simulink model "Segway_NL_nuovip"  (R2023b)
settings: Solver=ode1be  StartTime=0.0  StopTime=50  RelTol=1e-3
values from neighbouring files (symbols this model uses):
  dphi_0 = 0    [Parametri_Segway_Simulink_CSI_nuovip.m]
  dtheta_0 = 0    [Parametri_Segway_Simulink_CSI_nuovip.m]
  dx_0 = 0    [Parametri_Segway_Simulink_CSI_nuovip.m]
  Ga_nom_ss = minreal(Ga_nom_ss)    [CSI1_Segway_LQG_nuovip.m]
  K_LQG = -lqgreg(kest, Klqr)    [CSI1_Segway_LQG_nuovip.m]
  phi_0 = 0*pi/180    (= 0)    [Parametri_Segway_Simulink_CSI_nuovip.m]
  theta_0 = 0    [Parametri_Segway_Simulink_CSI_nuovip.m]
  x_0 = 0    [Parametri_Segway_Simulink_CSI_nuovip.m]
undefined symbols (not defined in the file or in its folder): K_DK, K_MS
settings Model: Creator=dario  LastModifiedBy=dario
settings OptimizationCC: ReuseModelBlockBuffer=off

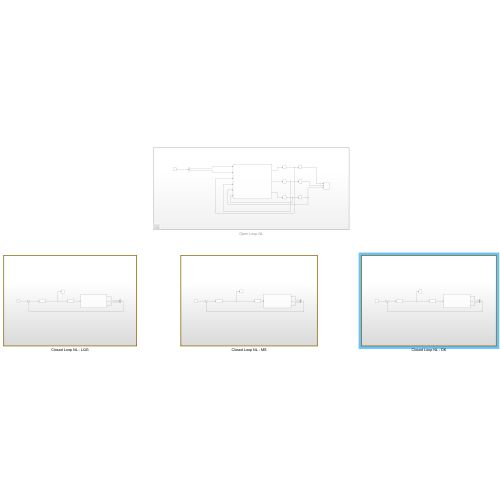
[thumbnail: Simulink's stored preview of the top-level diagram]
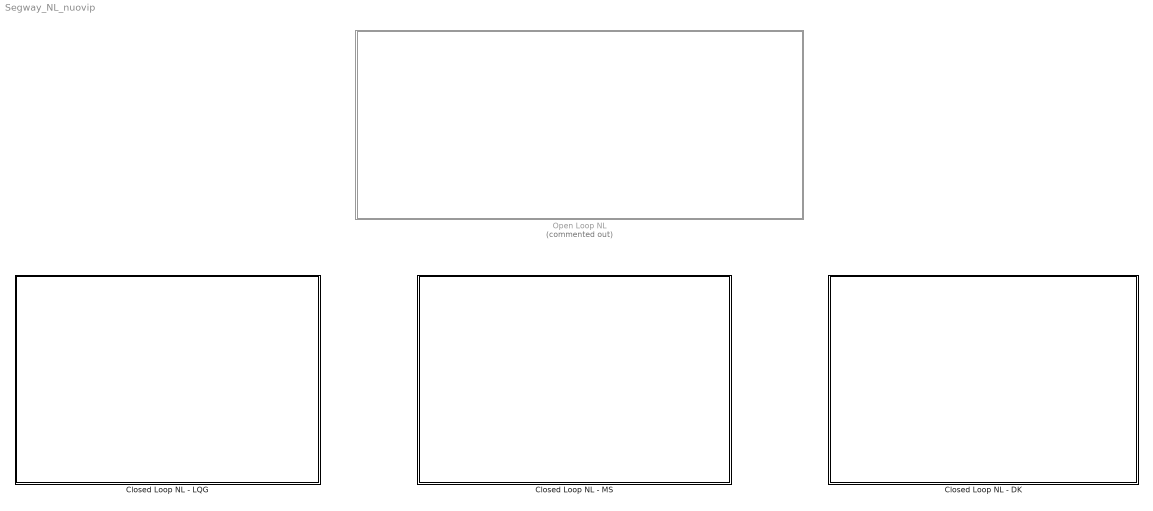
== system Segway_NL_nuovip ==
  Closed Loop NL - DK : Subsystem
  Closed Loop NL - LQG : Subsystem
  Closed Loop NL - MS : Subsystem
  Open Loop NL : Subsystem  Commented=on

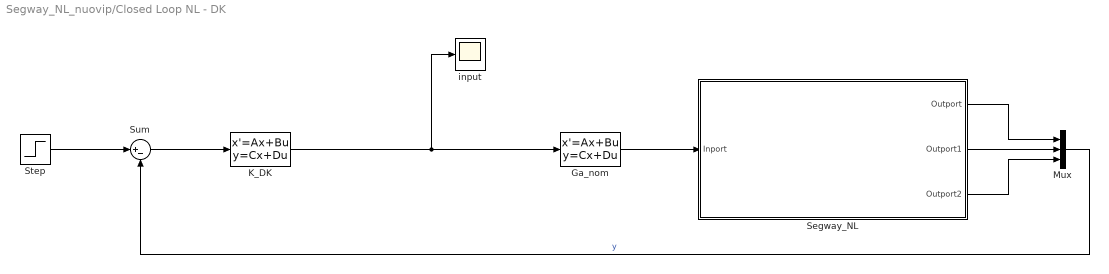
== system Segway_NL_nuovip/Closed Loop NL - DK ==
  Ga_nom : StateSpace  A=Ga_nom_ss.A  B=Ga_nom_ss.B  C=Ga_nom_ss.C  D=Ga_nom_ss.D  InitialCondition=0
  K_DK : StateSpace  A=K_DK.A  B=K_DK.B  C=K_DK.C  D=K_DK.D  InitialCondition=0
  Mux : Mux  Inputs=3
  Segway_NL : Subsystem
  Step : Step  Time=5  Before=[0 0 0]'  After=[0.1 0 0]'  SampleTime=0
  Sum : Sum  Inputs=|+-
  input : Scope
  wires:
  Segway_NL/3(Outport2) -> Mux/3
  K_DK/1 -> Ga_nom/1, input/1
  Step/1 -> Sum/1
  Mux/1 -> Sum/2  "y"
  Ga_nom/1 -> Segway_NL/1(Inport)
  Segway_NL/2(Outport1) -> Mux/2
  Segway_NL/1(Outport) -> Mux/1
  Sum/1 -> K_DK/1

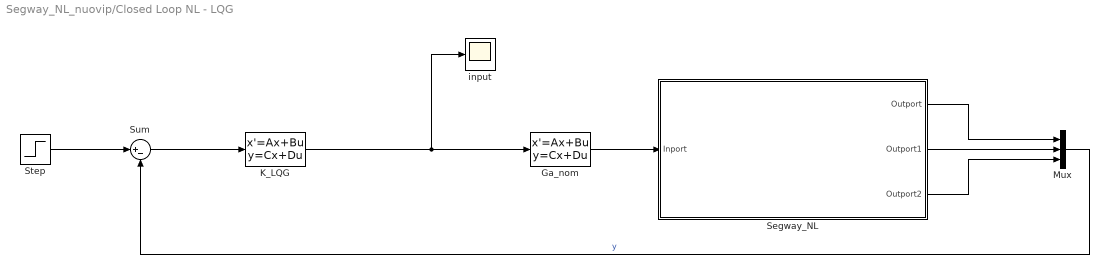
== system Segway_NL_nuovip/Closed Loop NL - LQG ==
  Ga_nom : StateSpace  A=Ga_nom_ss.A  B=Ga_nom_ss.B  C=Ga_nom_ss.C  D=Ga_nom_ss.D  InitialCondition=0
  K_LQG : StateSpace  A=K_LQG.A  B=K_LQG.B  C=K_LQG.C  D=K_LQG.D  InitialCondition=0
  Mux : Mux  Inputs=3
  Segway_NL : Subsystem
  Step : Step  Time=5  Before=[0 0 0]'  After=[10 0 0]'  SampleTime=0
  Sum : Sum  Inputs=|+-
  input : Scope
  wires:
  Segway_NL/3(Outport2) -> Mux/3
  K_LQG/1 -> Ga_nom/1, input/1
  Step/1 -> Sum/1
  Mux/1 -> Sum/2  "y"
  Ga_nom/1 -> Segway_NL/1(Inport)
  Segway_NL/2(Outport1) -> Mux/2
  Segway_NL/1(Outport) -> Mux/1
  Sum/1 -> K_LQG/1

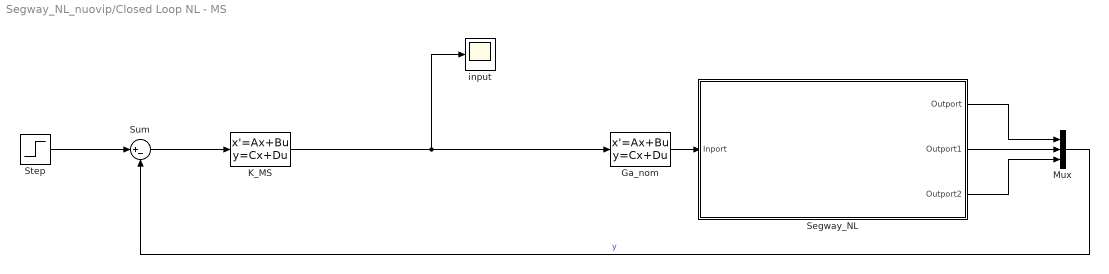
== system Segway_NL_nuovip/Closed Loop NL - MS ==
  Ga_nom : StateSpace  A=Ga_nom_ss.A  B=Ga_nom_ss.B  C=Ga_nom_ss.C  D=Ga_nom_ss.D  InitialCondition=0
  K_MS : StateSpace  A=K_MS.A  B=K_MS.B  C=K_MS.C  D=K_MS.D  InitialCondition=0
  Mux : Mux  Inputs=3
  Segway_NL : Subsystem
  Step : Step  Time=2  Before=[0 0 0]'  After=[50 0 0]'  SampleTime=0
  Sum : Sum  Inputs=|+-
  input : Scope
  wires:
  Sum/1 -> K_MS/1
  Segway_NL/1(Outport) -> Mux/1
  Segway_NL/2(Outport1) -> Mux/2
  Ga_nom/1 -> Segway_NL/1(Inport)
  Mux/1 -> Sum/2  "y"
  Step/1 -> Sum/1
  K_MS/1 -> input/1, Ga_nom/1
  Segway_NL/3(Outport2) -> Mux/3

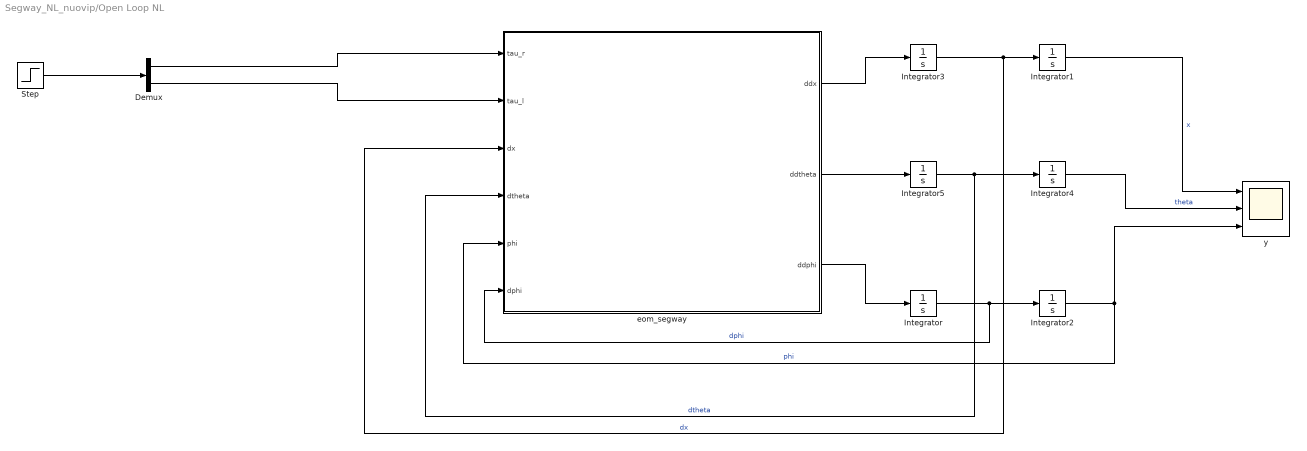
== system Segway_NL_nuovip/Open Loop NL ==
  Demux : Demux  Outputs=2
  Integrator : Integrator  InitialCondition=dphi_0
  Integrator1 : Integrator  InitialCondition=x_0
  Integrator2 : Integrator  InitialCondition=phi_0
  Integrator3 : Integrator  InitialCondition=dx_0
  Integrator4 : Integrator  InitialCondition=theta_0
  Integrator5 : Integrator  InitialCondition=dtheta_0
  Step : Step  Time=5  Before=[0 0]'  After=0.01*[1 1]'  SampleTime=0
  eom_segway : MATLAB Function  TreatAsAtomicUnit=on
  y : Scope  NumInputPorts=3
  wires:
  Integrator1/1 -> y/1  "x"
  Integrator4/1 -> y/2  "theta"
  Integrator5/1 -> eom_segway/4(dtheta), Integrator4/1  "dtheta"
  Demux/1 -> eom_segway/1(tau_r)
  Demux/2 -> eom_segway/2(tau_l)
  eom_segway/3(ddphi) -> Integrator/1
  Integrator3/1 -> eom_segway/3(dx), Integrator1/1  "dx"
  Integrator2/1 -> y/3, eom_segway/5(phi)  "phi"
  eom_segway/1(ddx) -> Integrator3/1
  Integrator/1 -> eom_segway/6(dphi), Integrator2/1  "dphi"
  eom_segway/2(ddtheta) -> Integrator5/1
  Step/1 -> Demux/1

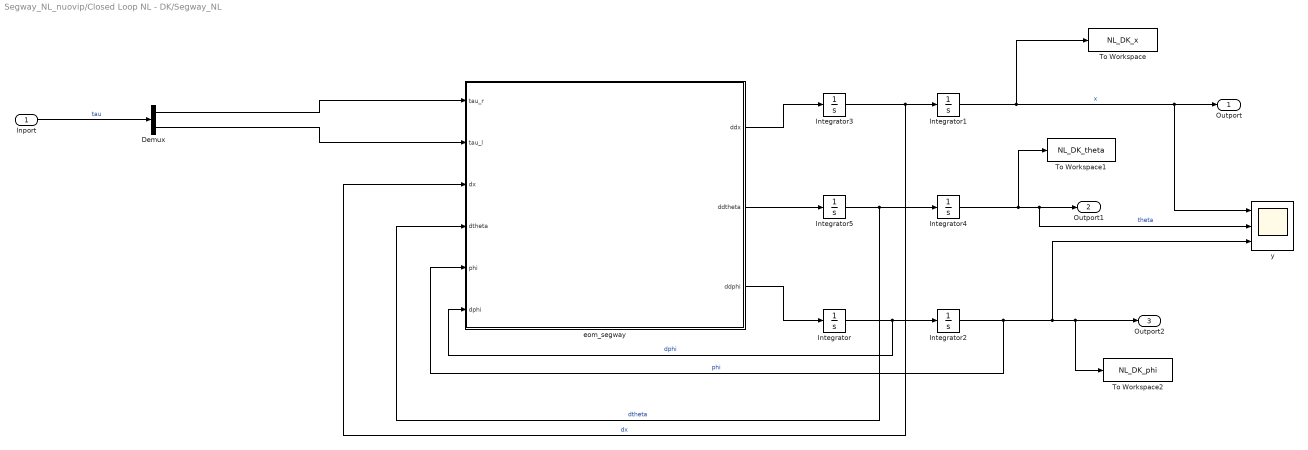
== system Segway_NL_nuovip/Closed Loop NL - DK/Segway_NL ==
  Inport : Inport
  Demux : Demux  Outputs=2
  Integrator : Integrator  InitialCondition=dphi_0
  Integrator1 : Integrator  InitialCondition=x_0
  Integrator2 : Integrator  InitialCondition=phi_0
  Integrator3 : Integrator  InitialCondition=dx_0
  Integrator4 : Integrator  InitialCondition=theta_0
  Integrator5 : Integrator  InitialCondition=dtheta_0
  To Workspace : ToWorkspace  VariableName=NL_DK_x  SaveFormat=Timeseries  SampleTime=-1
  To Workspace1 : ToWorkspace  VariableName=NL_DK_theta  SaveFormat=Timeseries  SampleTime=-1
  To Workspace2 : ToWorkspace  VariableName=NL_DK_phi  SaveFormat=Timeseries  SampleTime=-1
  eom_segway : MATLAB Function  TreatAsAtomicUnit=on
  y : Scope  NumInputPorts=3
  Outport : Outport
  Outport1 : Outport  Port=2
  Outport2 : Outport  Port=3
  wires:
  Integrator1/1 -> To Workspace/1, y/1, Outport/1  "x"
  eom_segway/1(ddx) -> Integrator3/1
  Integrator2/1 -> y/3, To Workspace2/1, Outport2/1, eom_segway/5(phi)  "phi"
  Integrator/1 -> eom_segway/6(dphi), Integrator2/1  "dphi"
  Integrator3/1 -> eom_segway/3(dx), Integrator1/1  "dx"
  eom_segway/3(ddphi) -> Integrator/1
  eom_segway/2(ddtheta) -> Integrator5/1
  Integrator5/1 -> eom_segway/4(dtheta), Integrator4/1  "dtheta"
  Integrator4/1 -> To Workspace1/1, y/2, Outport1/1  "theta"
  Inport/1 -> Demux/1  "tau"
  Demux/1 -> eom_segway/1(tau_r)
  Demux/2 -> eom_segway/2(tau_l)

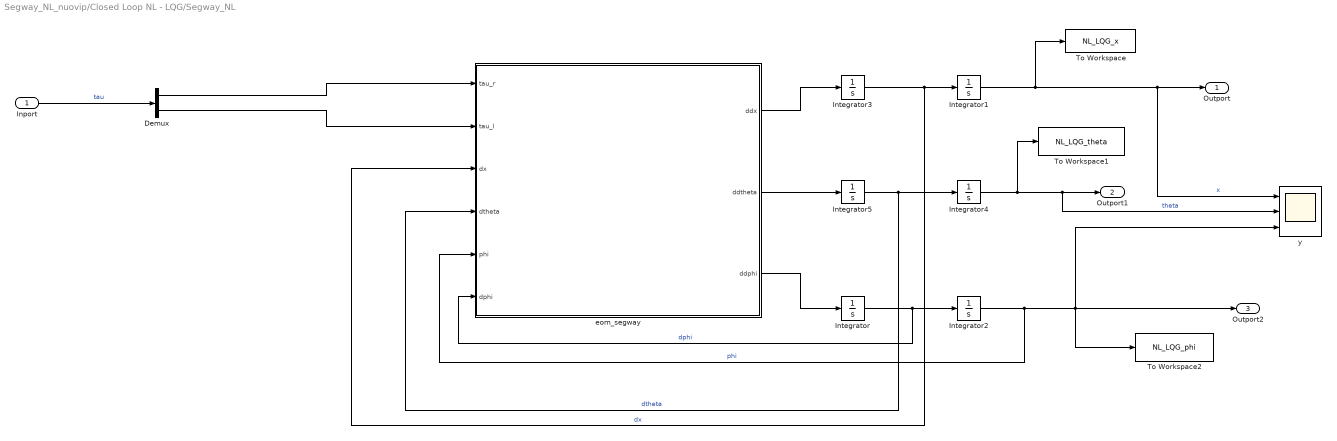
== system Segway_NL_nuovip/Closed Loop NL - LQG/Segway_NL ==
  Inport : Inport
  Demux : Demux  Outputs=2
  Integrator : Integrator  InitialCondition=dphi_0
  Integrator1 : Integrator  InitialCondition=x_0
  Integrator2 : Integrator  InitialCondition=phi_0
  Integrator3 : Integrator  InitialCondition=dx_0
  Integrator4 : Integrator  InitialCondition=theta_0
  Integrator5 : Integrator  InitialCondition=dtheta_0
  To Workspace : ToWorkspace  VariableName=NL_LQG_x  SaveFormat=Timeseries  SampleTime=-1
  To Workspace1 : ToWorkspace  VariableName=NL_LQG_theta  SaveFormat=Timeseries  SampleTime=-1
  To Workspace2 : ToWorkspace  VariableName=NL_LQG_phi  SaveFormat=Timeseries  SampleTime=-1
  eom_segway : MATLAB Function  TreatAsAtomicUnit=on
  y : Scope  NumInputPorts=3
  Outport : Outport
  Outport1 : Outport  Port=2
  Outport2 : Outport  Port=3
  wires:
  Integrator1/1 -> To Workspace/1, y/1, Outport/1  "x"
  eom_segway/1(ddx) -> Integrator3/1
  Integrator2/1 -> To Workspace2/1, y/3, Outport2/1, eom_segway/5(phi)  "phi"
  Integrator/1 -> eom_segway/6(dphi), Integrator2/1  "dphi"
  Integrator3/1 -> eom_segway/3(dx), Integrator1/1  "dx"
  eom_segway/3(ddphi) -> Integrator/1
  eom_segway/2(ddtheta) -> Integrator5/1
  Integrator5/1 -> eom_segway/4(dtheta), Integrator4/1  "dtheta"
  Integrator4/1 -> To Workspace1/1, y/2, Outport1/1  "theta"
  Inport/1 -> Demux/1  "tau"
  Demux/1 -> eom_segway/1(tau_r)
  Demux/2 -> eom_segway/2(tau_l)

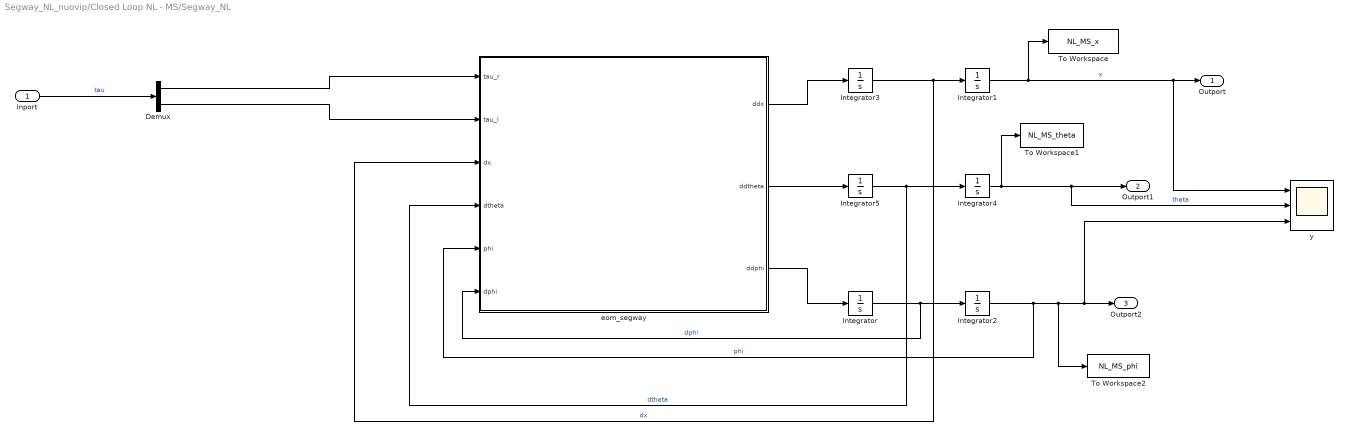
== system Segway_NL_nuovip/Closed Loop NL - MS/Segway_NL ==
  Inport : Inport
  Demux : Demux  Outputs=2
  Integrator : Integrator  InitialCondition=dphi_0
  Integrator1 : Integrator  InitialCondition=x_0
  Integrator2 : Integrator  InitialCondition=phi_0
  Integrator3 : Integrator  InitialCondition=dx_0
  Integrator4 : Integrator  InitialCondition=theta_0
  Integrator5 : Integrator  InitialCondition=dtheta_0
  To Workspace : ToWorkspace  VariableName=NL_MS_x  SaveFormat=Timeseries  SampleTime=-1
  To Workspace1 : ToWorkspace  VariableName=NL_MS_theta  SaveFormat=Timeseries  SampleTime=-1
  To Workspace2 : ToWorkspace  VariableName=NL_MS_phi  SaveFormat=Timeseries  SampleTime=-1
  eom_segway : MATLAB Function  TreatAsAtomicUnit=on
  y : Scope  NumInputPorts=3
  Outport : Outport
  Outport1 : Outport  Port=2
  Outport2 : Outport  Port=3
  wires:
  Demux/2 -> eom_segway/2(tau_l)
  Demux/1 -> eom_segway/1(tau_r)
  Inport/1 -> Demux/1  "tau"
  Integrator4/1 -> To Workspace1/1, Outport1/1, y/2  "theta"
  Integrator5/1 -> Integrator4/1, eom_segway/4(dtheta)  "dtheta"
  eom_segway/2(ddtheta) -> Integrator5/1
  eom_segway/3(ddphi) -> Integrator/1
  Integrator3/1 -> Integrator1/1, eom_segway/3(dx)  "dx"
  Integrator/1 -> Integrator2/1, eom_segway/6(dphi)  "dphi"
  Integrator2/1 -> eom_segway/5(phi), To Workspace2/1, Outport2/1, y/3  "phi"
  eom_segway/1(ddx) -> Integrator3/1
  Integrator1/1 -> To Workspace/1, Outport/1, y/1  "x"

== matlab function Segway_NL_nuovip/Open Loop NL/eom_segway ==
  data: ddx output size=1; ddtheta output; tau_r input; tau_l input; dx input; dtheta input; phi input; dphi input; ddphi output; eom_params parameter
% function that describes the EoM

function [ddx, ddtheta, ddphi] = eom_segway(tau_r, tau_l, dx, dtheta, phi, dphi, eom_params)

% rename the parameters inside the struct
r = eom_params.wheel_radius;
mb = eom_params.body_mass;
mw = eom_params.wheel_mass;
g = eom_params.gravity;
L = eom_params.center_of_mass;
a = eom_params.semiaxis_wheels;

% Operations in order to get the EoM
M_ddx = 2*(3/2*mw + 1/2*mb);
M_ddt = 2*(3/2*mw*a^2 + 1/6*mb*a^2 + 1/2*mb*L^2*sin(phi)^2);
M_ddp = 2*(1/2*mw*r^2 + 2/3*mb*L^2);

M_ddxp = -mw*r + mb*L*cos(phi);

C_dx = -mb*L*sin(phi)*(dphi^2 + dtheta^2);
C_dt = 2*mb*L^2*sin(phi)*cos(phi)*dtheta*dphi + mb*L*sin(phi)*dx*dtheta;
C_dp = -mb*L^2*sin(phi)*cos(phi)*dtheta^2;

g_p = -mb*g*L*sin(phi);

M = [M_ddx 0 M_ddxp;
     0 M_ddt 0;
     M_ddxp 0 M_ddp];
C = [C_dx C_dt C_dp]';
G = [0 0 g_p]';

C_tau = [1/r 1/r;
         a/r -a/r;
         -1 -1];

q = inv(M)*(-C -G + C_tau*[tau_r tau_l]'); % inv(M)*...

ddx = q(1);
ddtheta = q(2);
ddphi = q(3);

== matlab function Segway_NL_nuovip/Closed Loop NL - LQG/Segway_NL/eom_segway ==
  data: ddx output size=1; ddtheta output; tau_r input; tau_l input; dx input; dtheta input; phi input; dphi input; ddphi output; eom_params parameter
% function that describes the EoM

function [ddx, ddtheta, ddphi] = eom_segway(tau_r, tau_l, dx, dtheta, phi, dphi, eom_params)

% rename the parameters inside the struct
r = eom_params.wheel_radius;
mb = eom_params.body_mass;
mw = eom_params.wheel_mass;
g = eom_params.gravity;
L = eom_params.center_of_mass;
a = eom_params.semiaxis_wheels;

% Operations in order to get the EoM
M_ddx = 2*(3/2*mw + 1/2*mb);
M_ddt = 2*(3/2*mw*a^2 + 1/6*mb*a^2 + 1/2*mb*L^2*sin(phi)^2);
M_ddp = 2*(1/2*mw*r^2 + 2/3*mb*L^2);

M_ddxp = -mw*r + mb*L*cos(phi);

C_dx = -mb*L*sin(phi)*(dphi^2 + dtheta^2);
C_dt = 2*mb*L^2*sin(phi)*cos(phi)*dtheta*dphi + mb*L*sin(phi)*dx*dtheta;
C_dp = -mb*L^2*sin(phi)*cos(phi)*dtheta^2;

g_p = -mb*g*L*sin(phi);

M = [M_ddx 0 M_ddxp;
     0 M_ddt 0;
     M_ddxp 0 M_ddp];
C = [C_dx C_dt C_dp]';
G = [0 0 g_p]';

C_tau = [1/r 1/r;
         a/r -a/r;
         -1 -1];

q = M\(-C -G + C_tau*[tau_r tau_l]'); % inv(M)*...

ddx = q(1);
ddtheta = q(2);
ddphi = q(3);

== matlab function Segway_NL_nuovip/Closed Loop NL - MS/Segway_NL/eom_segway ==
  data: ddx output size=1; ddtheta output; tau_r input; tau_l input; dx input; dtheta input; phi input; dphi input; ddphi output; eom_params parameter
% function that describes the EoM

function [ddx, ddtheta, ddphi] = eom_segway(tau_r, tau_l, dx, dtheta, phi, dphi, eom_params)

% rename the parameters inside the struct
r = eom_params.wheel_radius;
mb = eom_params.body_mass;
mw = eom_params.wheel_mass;
g = eom_params.gravity;
L = eom_params.center_of_mass;
a = eom_params.semiaxis_wheels;

% Operations in order to get the EoM
M_ddx = 2*(3/2*mw + 1/2*mb);
M_ddt = 2*(3/2*mw*a^2 + 1/6*mb*a^2 + 1/2*mb*L^2*sin(phi)^2);
M_ddp = 2*(1/2*mw*r^2 + 2/3*mb*L^2);

M_ddxp = -mw*r + mb*L*cos(phi);

C_dx = -mb*L*sin(phi)*(dphi^2 + dtheta^2);
C_dt = 2*mb*L^2*sin(phi)*cos(phi)*dtheta*dphi + mb*L*sin(phi)*dx*dtheta;
C_dp = -mb*L^2*sin(phi)*cos(phi)*dtheta^2;

g_p = -mb*g*L*sin(phi);

M = [M_ddx 0 M_ddxp;
     0 M_ddt 0;
     M_ddxp 0 M_ddp];
C = [C_dx C_dt C_dp]';
G = [0 0 g_p]';

C_tau = [1/r 1/r;
         a/r -a/r;
         -1 -1];

q = M\(-C -G + C_tau*[tau_r tau_l]'); % inv(M)*...

ddx = q(1);
ddtheta = q(2);
ddphi = q(3);

== matlab function Segway_NL_nuovip/Closed Loop NL - DK/Segway_NL/eom_segway ==
  data: ddx output size=1; ddtheta output; tau_r input; tau_l input; dx input; dtheta input; phi input; dphi input; ddphi output; eom_params parameter
% function that describes the EoM

function [ddx, ddtheta, ddphi] = eom_segway(tau_r, tau_l, dx, dtheta, phi, dphi, eom_params)

% rename the parameters inside the struct
r = eom_params.wheel_radius;
mb = eom_params.body_mass;
mw = eom_params.wheel_mass;
g = eom_params.gravity;
L = eom_params.center_of_mass;
a = eom_params.semiaxis_wheels;

% Operations in order to get the EoM
M_ddx = 2*(3/2*mw + 1/2*mb);
M_ddt = 2*(3/2*mw*a^2 + 1/6*mb*a^2 + 1/2*mb*L^2*sin(phi)^2);
M_ddp = 2*(1/2*mw*r^2 + 2/3*mb*L^2);

M_ddxp = -mw*r + mb*L*cos(phi);

C_dx = -mb*L*sin(phi)*(dphi^2 + dtheta^2);
C_dt = 2*mb*L^2*sin(phi)*cos(phi)*dtheta*dphi + mb*L*sin(phi)*dx*dtheta;
C_dp = -mb*L^2*sin(phi)*cos(phi)*dtheta^2;

g_p = -mb*g*L*sin(phi);

M = [M_ddx 0 M_ddxp;
     0 M_ddt 0;
     M_ddxp 0 M_ddp];
C = [C_dx C_dt C_dp]';
G = [0 0 g_p]';

C_tau = [1/r 1/r;
         a/r -a/r;
         -1 -1];

q = M\(-C -G + C_tau*[tau_r tau_l]'); % inv(M)*...

ddx = q(1);
ddtheta = q(2);
ddphi = q(3);
